simulink model "RC_Circuit"  (R2015b)
settings: Solver=ode1  StartTime=0.0  StopTime=20.0  FixedStep=0.001  RelTol=1e-3
model workspace (MAT data in the model file):
  C = 0.001
  R = 1000
  V = 5
  ans = 1
settings Model: Creator=aemili  LastModifiedBy=aemili

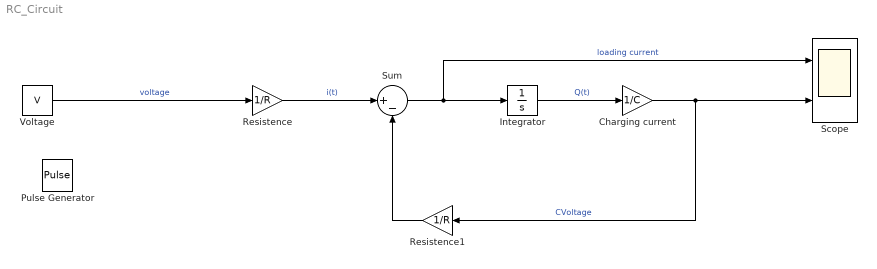
== system RC_Circuit ==
  Charging current : Gain  Gain=1/C
  Integrator : Integrator
  Pulse Generator : DiscretePulseGenerator  PulseType=Time based  Amplitude=5  Period=10  PulseWidth=50
  Resistence : Gain  Gain=1/R
  Resistence1 : Gain  Gain=1/R
  Scope : Scope  NumInputPorts=2
  Sum : Sum  Inputs=|+-
  Voltage : Constant  Value=V
  wires:
  Voltage/1 -> Resistence/1  "voltage"
  Resistence/1 -> Sum/1  "i(t)"
  Integrator/1 -> Charging current/1  "Q(t)"
  Charging current/1 -> Scope/2, Resistence1/1  "CVoltage"
  Sum/1 -> Scope/1, Integrator/1  "loading current"
  Resistence1/1 -> Sum/2
